simulink model "TestMassAccelerometer_LinearModel_LQR_Simulink2017"  (R2018b)
settings: Solver=ode4  StartTime=0.0  StopTime=SIM_TIME  FixedStep=STEP_SIZE  RelTol=1e-3
undefined symbols (not defined in the file): A0, A1, Aol, Bol, K_lqr_fs, K_lqr_int, STEP_TIME, Ts, x0, x0_int
settings Model: Creator=Roberto  LastModifiedBy=Roberto
settings SFSimCC: SimUseLocalCustomCode=off
settings RTWCC: RTWUseLocalCustomCode=off
settings CodeAppCC: StateflowObjectComments=on

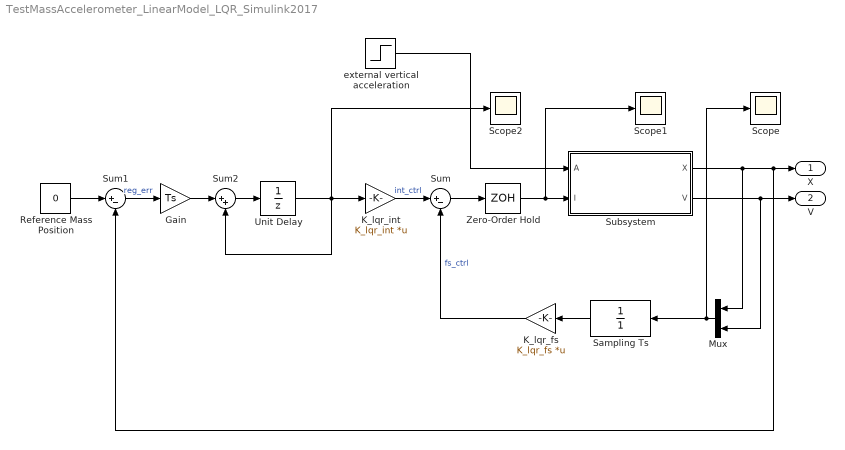
== system TestMassAccelerometer_LinearModel_LQR_Simulink2017 ==
  Gain : Gain  Gain=Ts
  K_lqr_fs : Gain  Gain=K_lqr_fs  Multiplication=Matrix(K*u)
  K_lqr_int : Gain  Gain=K_lqr_int  Multiplication=Matrix(K*u) (u vector)
  Mux : Mux  Inputs=2
  Reference Mass Position : Constant  Value=0
  Sampling Ts : DiscreteTransferFcn  Denominator=[1]  SampleTime=Ts
  Scope : Scope
  Scope1 : Scope
  Scope2 : Scope
  Subsystem : Subsystem
  Sum : Sum  Inputs=|+-
  Sum1 : Sum  Inputs=|+-
  Sum2 : Sum  Inputs=|++
  Unit Delay : UnitDelay  InitialCondition=x0_int  SampleTime=Ts
  Zero-Order Hold : ZeroOrderHold  SampleTime=Ts
  external vertical acceleration : Step  Time=STEP_TIME  Before=A0  After=A1  SampleTime=0
  X : Outport
  V : Outport  Port=2
  wires:
  Reference Mass Position/1 -> Sum1/1
  Sum/1 -> Zero-Order Hold/1
  Subsystem/2(V) -> Mux/2, V/1
  Mux/1 -> Sampling Ts/1, Scope/1
  K_lqr_fs/1 -> Sum/2  "fs_ctrl"
  Unit Delay/1 -> Scope2/1, Sum2/2, K_lqr_int/1
  Subsystem/1(X) -> Mux/1, Sum1/2, X/1
  K_lqr_int/1 -> Sum/1  "int_ctrl"
  Sum1/1 -> Gain/1  "reg_err"
  Sum2/1 -> Unit Delay/1
  external vertical acceleration/1 -> Subsystem/1(A)
  Sampling Ts/1 -> K_lqr_fs/1
  Zero-Order Hold/1 -> Scope1/1, Subsystem/2(I)
  Gain/1 -> Sum2/1

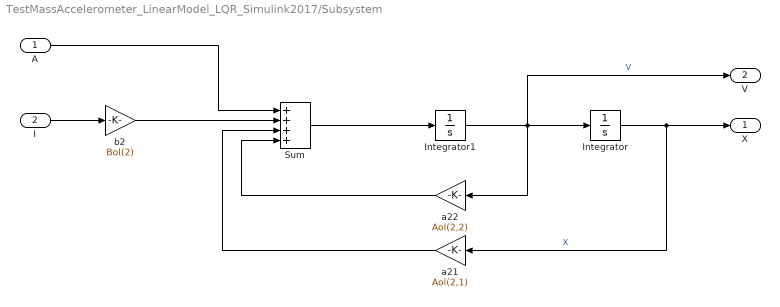
== system TestMassAccelerometer_LinearModel_LQR_Simulink2017/Subsystem ==
  A : Inport
  I : Inport  Port=2
  Integrator : Integrator  Priority=1  InitialCondition=x0(1)
  Integrator1 : Integrator  Priority=2  InitialCondition=x0(2)
  Sum : Sum  Inputs=++++
  a21 : Gain  Gain=Aol(2,1)
  a22 : Gain  Gain=Aol(2,2)
  b2 : Gain  Gain=Bol(2)
  X : Outport
  V : Outport  Port=2
  wires:
  Integrator1/1 -> a22/1, V/1, Integrator/1  "V"
  Sum/1 -> Integrator1/1
  A/1 -> Sum/1
  Integrator/1 -> a21/1, X/1  "X"
  a22/1 -> Sum/4
  a21/1 -> Sum/3
  I/1 -> b2/1
  b2/1 -> Sum/2
